simulink model "crazyflie_ros"  (R2021a)
settings: Solver=FixedStepAuto  StartTime=0.0  StopTime=inf  FixedStep=0.01  RelTol=1e-3
libraries: robotlib x5, aerolibconvert2 x3, sharedtransform x3
settings Model: Creator=julio  LastModifiedBy=julio

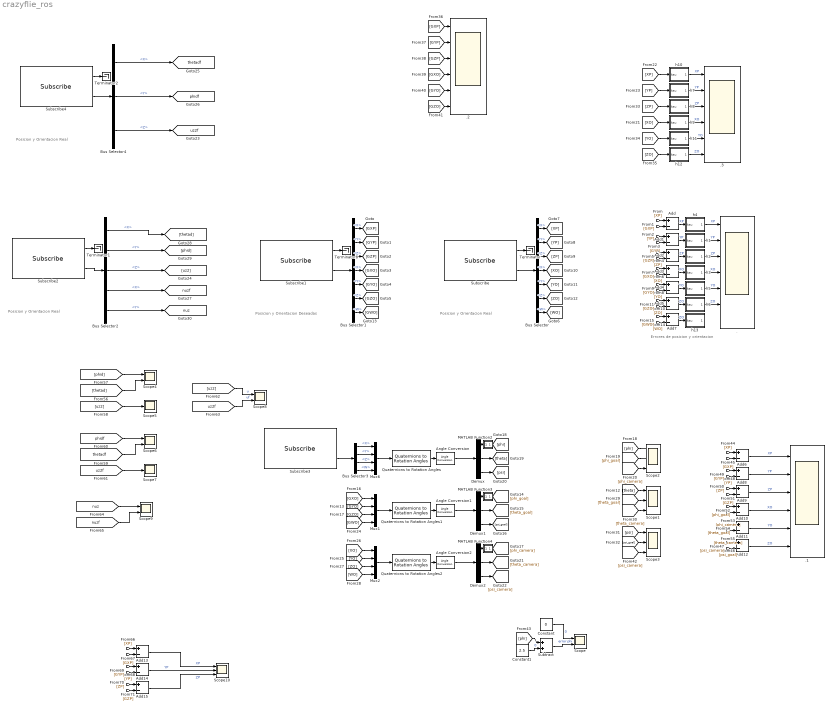
== system crazyflie_ros ==
  note: Posicion y Orientacion Deseadas
  note: Posicion y Orientacion Real
  note: Errores de posicion y orientacion
  note: Posicion y Orientacion Real
  note: Posicion y Orientacion Real
  . : Scope  NumInputPorts=7
  .1 : Scope  NumInputPorts=6
  .2 : Scope  NumInputPorts=6
  .3 : Scope  NumInputPorts=6
  Add{,1..15} (16 alike) : Sum  Inputs=+-
  Angle Conversion : aerolibconvert2/Angle Conversion  IU=rad  OU=deg
  Angle Conversion1 : aerolibconvert2/Angle Conversion  IU=rad  OU=deg
  Angle Conversion2 : aerolibconvert2/Angle Conversion  IU=rad  OU=deg
  Bus Selector : BusSelector  OutputSignals=Pose.Position.X,Pose.Position.Y,Pose.Position.Z,Pose.Orientation.X,Pose.Orientation.Y,Pose.Orientation.Z,Pose.Orientation.W
  Bus Selector1 : BusSelector  OutputSignals=Pose.Position.X,Pose.Position.Y,Pose.Position.Z,Pose.Orientation.X,Pose.Orientation.Y,Pose.Orientation.Z,Pose.Orientation.W
  Bus Selector2 : BusSelector  OutputSignals=Linear.X,Linear.Y,Linear.Z,Angular.X,Angular.Y
  Bus Selector3 : BusSelector  OutputSignals=Pose.Orientation.X,Pose.Orientation.Y,Pose.Orientation.Z,Pose.Orientation.W
  Bus Selector4 : BusSelector  OutputSignals=Linear.X,Linear.Y,Linear.Z
  Constant : Constant  Value=0
  Constant1 : Constant  Value=2.5
  Demux : Demux  Outputs=3
  Demux1 : Demux  Outputs=3
  Demux2 : Demux  Outputs=3
  MATLAB Function2 : MATLAB Function  TreatAsAtomicUnit=on
  MATLAB Function3 : MATLAB Function  TreatAsAtomicUnit=on
  MATLAB Function4 : MATLAB Function  TreatAsAtomicUnit=on
  Mux1 : Mux
  Mux2 : Mux
  Mux6 : Mux
  Quaternions to Rotation Angles : sharedtransform/Quaternions to Rotation Angles  rotationOrder=ZYX  aMode=aMode
      settings: SourceProductBaseCode=AE,PW,DR,MT,UV,VE
  Quaternions to Rotation Angles1 : sharedtransform/Quaternions to Rotation Angles  rotationOrder=ZYX  aMode=aMode
      settings: SourceProductBaseCode=AE,PW,DR,MT,UV,VE
  Quaternions to Rotation Angles2 : sharedtransform/Quaternions to Rotation Angles  rotationOrder=ZYX  aMode=aMode
      settings: SourceProductBaseCode=AE,PW,DR,MT,UV,VE
  Scope{,4,6,8..9} (5 alike) : Scope  NumInputPorts=2
  Scope{1..3,10} (4 alike) : Scope  NumInputPorts=3
  Scope5 : Scope
  Scope7 : Scope
  Subscribe : robotlib/Subscribe  topicSource=Select from ROS network  topic=/crazyflie/vrpn_client_node/crazyflie/pose  messageType=geometry_msgs/PoseStamped  SampleTime=-1  legacyBusStruct=off  messageQueueLength=1
  Subscribe1 : robotlib/Subscribe  topicSource=Select from ROS network  topic=/crazyflie/goal  messageType=geometry_msgs/PoseStamped  SampleTime=-1  legacyBusStruct=off  messageQueueLength=1
  Subscribe2 : robotlib/Subscribe  topicSource=Select from ROS network  topic=/crazyflie/cmd_vel  messageType=geometry_msgs/Twist  SampleTime=-1  legacyBusStruct=off  messageQueueLength=1
  Subscribe3 : robotlib/Subscribe  topicSource=Select from ROS network  topic=/crazyflie/pose  messageType=geometry_msgs/PoseStamped  SampleTime=-1  legacyBusStruct=off  messageQueueLength=1
  Subscribe4 : robotlib/Subscribe  topicSource=Select from ROS network  topic=/crazyflie/filtered_cmd_vel  messageType=geometry_msgs/Twist  SampleTime=-1  legacyBusStruct=off  messageQueueLength=1
  Subtract : Sum
  Terminator{,1..2,8} (4 alike) : Terminator
  h1 : Subsystem
  h10 : Subsystem
  h11 : Subsystem
  h12 : Subsystem
  h13 : Subsystem
  h2 : Subsystem
  h3 : Subsystem
  h4 : Subsystem
  h5 : Subsystem
  h6 : Subsystem
  h7 : Subsystem
  h8 : Subsystem
  h9 : Subsystem
  tag scope: nuz=global, nuzf=global, phidf=global, thetadf=global, uz2f=global
  wires:
  Subscribe/1 -> Terminator/1
  Subscribe/2 -> Bus Selector/1
  Subscribe1/1 -> Terminator8/1
  Subscribe1/2 -> Bus Selector1/1
  Bus Selector1/1 -> [GXP]  "<X>"
  Bus Selector1/2 -> [GYP]  "<Y>"
  Bus Selector1/3 -> [GZP]  "<Z>"
  Bus Selector1/4 -> [GXO]  "<X>"
  Bus Selector1/5 -> [GYO]  "<Y>"
  Bus Selector1/6 -> [GZO]  "<Z>"
  Bus Selector/1 -> [XP]  "<X>"
  Bus Selector/3 -> [ZP]  "<Z>"
  Bus Selector/4 -> [XO]  "<X>"
  Bus Selector/2 -> [YP]  "<Y>"
  Bus Selector/5 -> [YO]  "<Y>"
  Bus Selector/6 -> [ZO]  "<Z>"
  h4/1(Out1) -> ./1  "XP"
  h1/1(Out1) -> ./2  "YP"
  h2/1(Out1) -> ./3  "ZP"
  h3/1(Out1) -> ./4  "XO"
  h5/1(Out1) -> ./5  "YO"
  h6/1(Out1) -> ./6  "ZO"
  [XP] -> Add/1
  [GXP] -> Add/2
  [GYP] -> Add1/2
  [YP] -> Add1/1
  [GZP] -> Add2/2
  [ZP] -> Add2/1
  [GXO] -> Add3/2
  [XO] -> Add3/1
  [GYO] -> Add4/2
  [YO] -> Add4/1
  [GZO] -> Add5/2
  [ZO] -> Add5/1
  Subscribe3/2 -> Bus Selector3/1
  Bus Selector3/1 -> Mux6/1  "<X>"
  Mux6/1 -> Quaternions to Rotation Angles/1
  Bus Selector3/2 -> Mux6/2  "<Y>"
  Bus Selector3/3 -> Mux6/3  "<Z>"
  Bus Selector3/4 -> Mux6/4  "<W>"
  [phi_camera] -> Scope2/3
  Quaternions to Rotation Angles/1 -> Angle Conversion/1
  Angle Conversion/1 -> Demux/1
  Demux/2 -> [theta]
  Demux/3 -> [psi]
  Add/1 -> h4/1(tau)  "XP"
  Add1/1 -> h1/1(tau)  "YP"
  Add2/1 -> h2/1(tau)  "ZP"
  Add3/1 -> h3/1(tau)  "XO"
  Add4/1 -> h5/1(tau)  "YO"
  Add5/1 -> h6/1(tau)  "ZO"
  [XO] -> h9/1(tau)
  [XP] -> h10/1(tau)
  [YP] -> h7/1(tau)
  [ZP] -> h8/1(tau)
  [YO] -> h11/1(tau)
  [ZO] -> h12/1(tau)
  [GXP] -> .2/1
  [GYP] -> .2/2
  [GZP] -> .2/3
  [GXO] -> .2/4
  [GYO] -> .2/5
  [GZO] -> .2/6
  h12/1(Out1) -> .3/6  "ZO"
  h11/1(Out1) -> .3/5  "YO"
  h9/1(Out1) -> .3/4  "XO"
  h8/1(Out1) -> .3/3  "ZP"
  h7/1(Out1) -> .3/2  "YP"
  h10/1(Out1) -> .3/1  "XP"
  Bus Selector/7 -> [WO]  "<W>"
  Bus Selector1/7 -> [GWO]  "<W>"
  [WO] -> Add7/1
  [GWO] -> Add7/2
  Add7/1 -> h13/1(tau)  "ZO"
  Demux1/3 -> [psi_goal]
  Demux1/2 -> [theta_goal]
  Angle Conversion1/1 -> Demux1/1
  Quaternions to Rotation Angles1/1 -> Angle Conversion1/1
  Mux1/1 -> Quaternions to Rotation Angles1/1
  [GXO] -> Mux1/1
  [GYO] -> Mux1/2
  [GZO] -> Mux1/3
  [GWO] -> Mux1/4
  [WO] -> Mux2/4
  [ZO] -> Mux2/3
  [YO] -> Mux2/2
  [XO] -> Mux2/1
  Mux2/1 -> Quaternions to Rotation Angles2/1
  Quaternions to Rotation Angles2/1 -> Angle Conversion2/1
  Angle Conversion2/1 -> Demux2/1
  Demux2/2 -> [theta_camera]
  [theta] -> Scope1/1
  [theta_camera] -> Scope1/3
  [theta_goal] -> Scope1/2
  [phi] -> Scope2/1
  [phi_goal] -> Scope2/2
  Demux/1 -> MATLAB Function2/1(phi)
  MATLAB Function2/1(phifilter) -> [phi]
  Demux1/1 -> MATLAB Function3/1(phi)
  MATLAB Function3/1(phifilter) -> [phi_goal]
  Demux2/1 -> MATLAB Function4/1(phi)
  MATLAB Function4/1(phifilter) -> [phi_camera]
  Demux2/3 -> [psi_camera]
  [phi] -> Subtract/1
  Subtract/1 -> Scope/2  "error phi"
  Constant/1 -> Scope/1  "0"
  Constant1/1 -> Subtract/2  "0"
  [psi] -> Scope3/1
  [psi_goal] -> Scope3/2
  [psi_camera] -> Scope3/3
  Add12/1 -> .1/6  "ZO"
  [XP] -> Add6/1
  [phi_camera] -> Add10/2
  Add10/1 -> .1/4  "XO"
  [phi_goal] -> Add10/1
  Add6/1 -> .1/1  "XP"
  [psi_goal] -> Add12/1
  [ZP] -> Add9/1
  [psi_camera] -> Add12/2
  [GXP] -> Add6/2
  [GZP] -> Add9/2
  [YP] -> Add8/1
  [GYP] -> Add8/2
  Add9/1 -> .1/3  "ZP"
  [theta_camera] -> Add11/2
  [theta_goal] -> Add11/1
  Add11/1 -> .1/5  "YO"
  Add8/1 -> .1/2  "YP"
  Subscribe2/2 -> Bus Selector2/1
  Subscribe2/1 -> Terminator1/1
  Bus Selector2/1 -> [thetad]  "<X>"
  Bus Selector2/3 -> [uz2]  "<Z>"
  Bus Selector2/2 -> [phid]  "<Y>"
  [phid] -> Scope4/1
  [thetad] -> Scope4/2
  [uz2] -> Scope5/1
  Bus Selector4/1 -> [thetadf]  "<X>"
  Bus Selector4/3 -> [uz2f]  "<Z>"
  Subscribe4/2 -> Bus Selector4/1
  Subscribe4/1 -> Terminator2/1
  Bus Selector4/2 -> [phidf]  "<Y>"
  [phidf] -> Scope6/1
  [thetadf] -> Scope6/2
  [uz2f] -> Scope7/1
  [uz2] -> Scope8/1  "u"
  [uz2f] -> Scope8/2  "uf"
  Bus Selector2/4 -> [nuzf]  "<X>"
  [nuz] -> Scope9/1
  Bus Selector2/5 -> [nuz]  "<Y>"
  [nuzf] -> Scope9/2
  Add15/1 -> Scope10/3  "ZP"
  Add14/1 -> Scope10/2  "YP"
  [ZP] -> Add15/1
  [GYP] -> Add14/2
  [XP] -> Add13/1
  [YP] -> Add14/1
  Add13/1 -> Scope10/1  "XP"
  [GZP] -> Add15/2
  [GXP] -> Add13/2

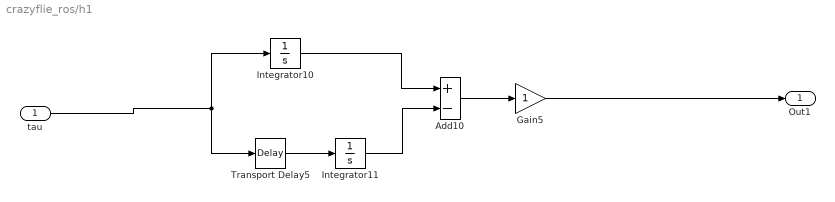
== system crazyflie_ros/h1 ==
  tau : Inport
  Add10 : Sum  Inputs=+-
  Gain5 : Gain
  Integrator10 : Integrator
  Integrator11 : Integrator
  Transport Delay5 : TransportDelay  BufferSize=2048
  Out1 : Outport  VectorParamsAs1DForOutWhenUnconnected=off
  wires:
  Add10/1 -> Gain5/1
  Gain5/1 -> Out1/1
  Integrator11/1 -> Add10/2
  Integrator10/1 -> Add10/1
  Transport Delay5/1 -> Integrator11/1
  tau/1 -> Transport Delay5/1, Integrator10/1

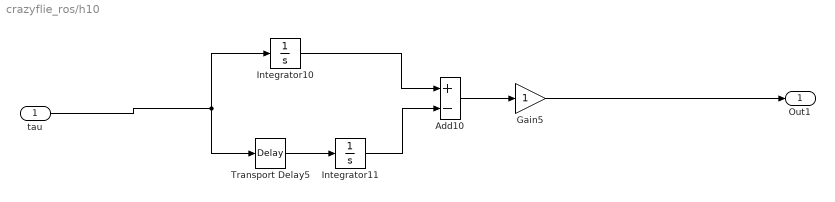
== system crazyflie_ros/h10 ==
  tau : Inport
  Add10 : Sum  Inputs=+-
  Gain5 : Gain
  Integrator10 : Integrator
  Integrator11 : Integrator
  Transport Delay5 : TransportDelay  BufferSize=2048
  Out1 : Outport  VectorParamsAs1DForOutWhenUnconnected=off
  wires:
  Add10/1 -> Gain5/1
  Gain5/1 -> Out1/1
  Integrator11/1 -> Add10/2
  Integrator10/1 -> Add10/1
  Transport Delay5/1 -> Integrator11/1
  tau/1 -> Transport Delay5/1, Integrator10/1

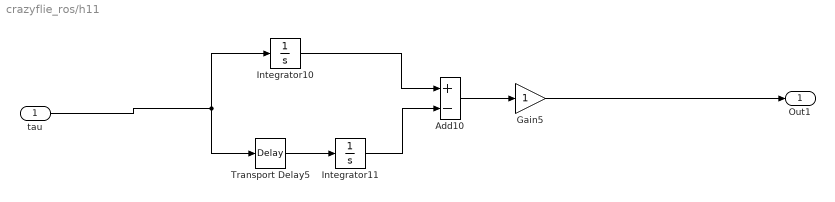
== system crazyflie_ros/h11 ==
  tau : Inport
  Add10 : Sum  Inputs=+-
  Gain5 : Gain
  Integrator10 : Integrator
  Integrator11 : Integrator
  Transport Delay5 : TransportDelay  BufferSize=2048
  Out1 : Outport  VectorParamsAs1DForOutWhenUnconnected=off
  wires:
  Add10/1 -> Gain5/1
  Gain5/1 -> Out1/1
  Integrator11/1 -> Add10/2
  Integrator10/1 -> Add10/1
  Transport Delay5/1 -> Integrator11/1
  tau/1 -> Transport Delay5/1, Integrator10/1

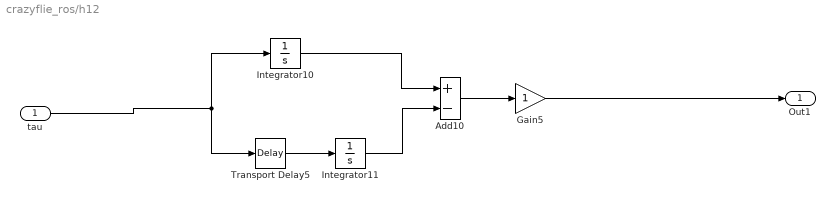
== system crazyflie_ros/h12 ==
  tau : Inport
  Add10 : Sum  Inputs=+-
  Gain5 : Gain
  Integrator10 : Integrator
  Integrator11 : Integrator
  Transport Delay5 : TransportDelay  BufferSize=2048
  Out1 : Outport  VectorParamsAs1DForOutWhenUnconnected=off
  wires:
  tau/1 -> Integrator10/1, Transport Delay5/1
  Transport Delay5/1 -> Integrator11/1
  Integrator10/1 -> Add10/1
  Integrator11/1 -> Add10/2
  Gain5/1 -> Out1/1
  Add10/1 -> Gain5/1

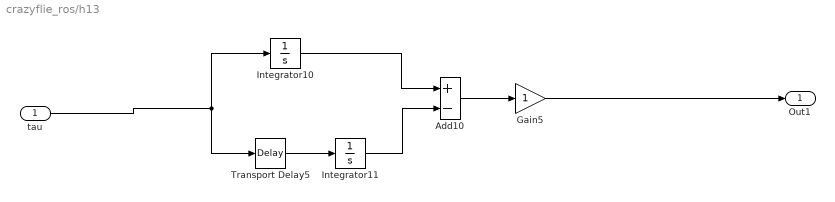
== system crazyflie_ros/h13 ==
  tau : Inport
  Add10 : Sum  Inputs=+-
  Gain5 : Gain
  Integrator10 : Integrator
  Integrator11 : Integrator
  Transport Delay5 : TransportDelay  BufferSize=2048
  Out1 : Outport  VectorParamsAs1DForOutWhenUnconnected=off
  wires:
  Add10/1 -> Gain5/1
  Gain5/1 -> Out1/1
  Integrator11/1 -> Add10/2
  Integrator10/1 -> Add10/1
  Transport Delay5/1 -> Integrator11/1
  tau/1 -> Transport Delay5/1, Integrator10/1

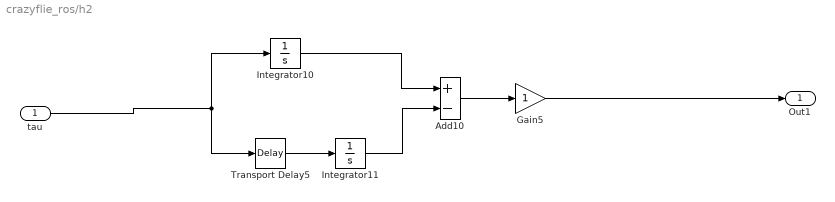
== system crazyflie_ros/h2 ==
  tau : Inport
  Add10 : Sum  Inputs=+-
  Gain5 : Gain
  Integrator10 : Integrator
  Integrator11 : Integrator
  Transport Delay5 : TransportDelay  BufferSize=2048
  Out1 : Outport  VectorParamsAs1DForOutWhenUnconnected=off
  wires:
  tau/1 -> Integrator10/1, Transport Delay5/1
  Transport Delay5/1 -> Integrator11/1
  Integrator10/1 -> Add10/1
  Integrator11/1 -> Add10/2
  Gain5/1 -> Out1/1
  Add10/1 -> Gain5/1

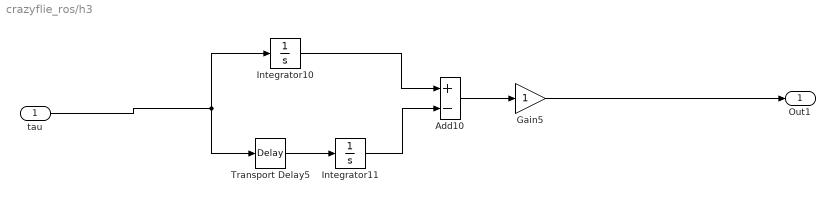
== system crazyflie_ros/h3 ==
  tau : Inport
  Add10 : Sum  Inputs=+-
  Gain5 : Gain
  Integrator10 : Integrator
  Integrator11 : Integrator
  Transport Delay5 : TransportDelay  BufferSize=2048
  Out1 : Outport  VectorParamsAs1DForOutWhenUnconnected=off
  wires:
  Add10/1 -> Gain5/1
  Gain5/1 -> Out1/1
  Integrator11/1 -> Add10/2
  Integrator10/1 -> Add10/1
  Transport Delay5/1 -> Integrator11/1
  tau/1 -> Transport Delay5/1, Integrator10/1

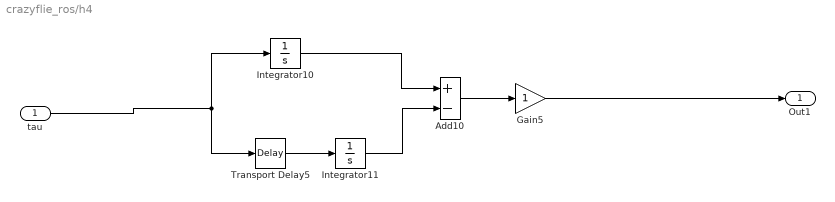
== system crazyflie_ros/h4 ==
  tau : Inport
  Add10 : Sum  Inputs=+-
  Gain5 : Gain
  Integrator10 : Integrator
  Integrator11 : Integrator
  Transport Delay5 : TransportDelay  BufferSize=2048
  Out1 : Outport  VectorParamsAs1DForOutWhenUnconnected=off
  wires:
  tau/1 -> Integrator10/1, Transport Delay5/1
  Transport Delay5/1 -> Integrator11/1
  Integrator10/1 -> Add10/1
  Integrator11/1 -> Add10/2
  Gain5/1 -> Out1/1
  Add10/1 -> Gain5/1

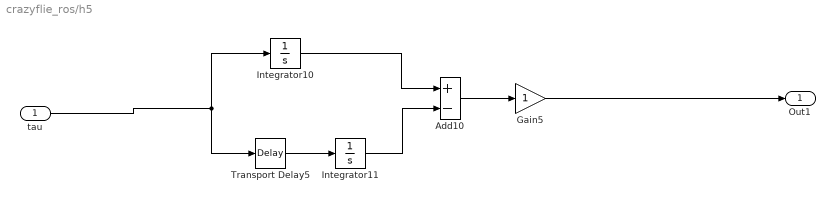
== system crazyflie_ros/h5 ==
  tau : Inport
  Add10 : Sum  Inputs=+-
  Gain5 : Gain
  Integrator10 : Integrator
  Integrator11 : Integrator
  Transport Delay5 : TransportDelay  BufferSize=2048
  Out1 : Outport  VectorParamsAs1DForOutWhenUnconnected=off
  wires:
  tau/1 -> Integrator10/1, Transport Delay5/1
  Transport Delay5/1 -> Integrator11/1
  Integrator10/1 -> Add10/1
  Integrator11/1 -> Add10/2
  Gain5/1 -> Out1/1
  Add10/1 -> Gain5/1

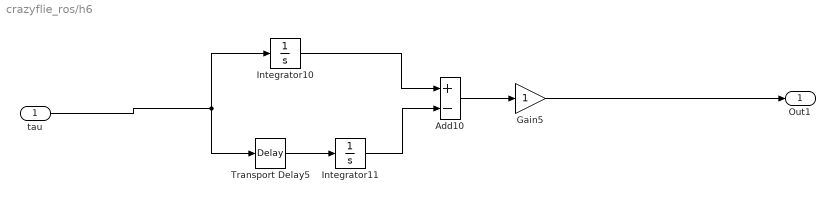
== system crazyflie_ros/h6 ==
  tau : Inport
  Add10 : Sum  Inputs=+-
  Gain5 : Gain
  Integrator10 : Integrator
  Integrator11 : Integrator
  Transport Delay5 : TransportDelay  BufferSize=2048
  Out1 : Outport  VectorParamsAs1DForOutWhenUnconnected=off
  wires:
  Add10/1 -> Gain5/1
  Gain5/1 -> Out1/1
  Integrator11/1 -> Add10/2
  Integrator10/1 -> Add10/1
  Transport Delay5/1 -> Integrator11/1
  tau/1 -> Transport Delay5/1, Integrator10/1

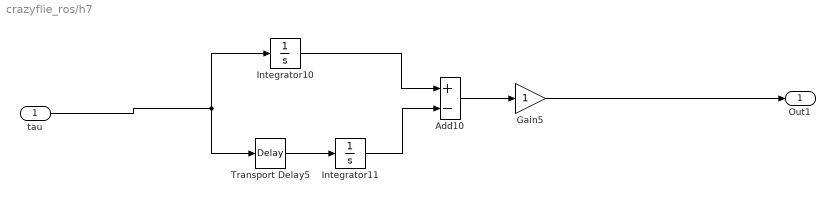
== system crazyflie_ros/h7 ==
  tau : Inport
  Add10 : Sum  Inputs=+-
  Gain5 : Gain
  Integrator10 : Integrator
  Integrator11 : Integrator
  Transport Delay5 : TransportDelay  BufferSize=2048
  Out1 : Outport  VectorParamsAs1DForOutWhenUnconnected=off
  wires:
  tau/1 -> Integrator10/1, Transport Delay5/1
  Transport Delay5/1 -> Integrator11/1
  Integrator10/1 -> Add10/1
  Integrator11/1 -> Add10/2
  Gain5/1 -> Out1/1
  Add10/1 -> Gain5/1

== system crazyflie_ros/h8 ==
  tau : Inport
  Add10 : Sum  Inputs=+-
  Gain5 : Gain
  Integrator10 : Integrator
  Integrator11 : Integrator
  Transport Delay5 : TransportDelay  BufferSize=2048
  Out1 : Outport  VectorParamsAs1DForOutWhenUnconnected=off
  wires:
  Add10/1 -> Gain5/1
  Gain5/1 -> Out1/1
  Integrator11/1 -> Add10/2
  Integrator10/1 -> Add10/1
  Transport Delay5/1 -> Integrator11/1
  tau/1 -> Transport Delay5/1, Integrator10/1

== system crazyflie_ros/h9 ==
  tau : Inport
  Add10 : Sum  Inputs=+-
  Gain5 : Gain
  Integrator10 : Integrator
  Integrator11 : Integrator
  Transport Delay5 : TransportDelay  BufferSize=2048
  Out1 : Outport  VectorParamsAs1DForOutWhenUnconnected=off
  wires:
  tau/1 -> Integrator10/1, Transport Delay5/1
  Transport Delay5/1 -> Integrator11/1
  Integrator10/1 -> Add10/1
  Integrator11/1 -> Add10/2
  Gain5/1 -> Out1/1
  Add10/1 -> Gain5/1

== matlab function crazyflie_ros/MATLAB Function3 ==
  data: phi input; phifilter output
function phifilter = fcn(phi)
lims=180;
limi=-180;
if phi<lims && phi>0
    phifilter=phi+limi;
elseif phi>limi && phi<0
    phifilter=phi+lims;
else
    phifilter=phi;
end

== matlab function crazyflie_ros/MATLAB Function4 ==
  data: phi input; phifilter output
function phifilter = fcn(phi)
lims=180;
limi=-180;
if phi<lims && phi>0
    phifilter=phi+limi;
elseif phi>limi && phi<0
    phifilter=phi+lims;
else
    phifilter=phi;
end

== matlab function crazyflie_ros/MATLAB Function2 ==
  data: phi input; phifilter output
function phifilter = fcn(phi)
lims=180;
limi=-180;
if phi<lims && phi>0
    phifilter=phi+limi;
elseif phi>limi && phi<0
    phifilter=phi+lims;
else
    phifilter=phi;
end
